simulink model "DC_motor_trans_fcn_25_04"  (R2020b)
settings: Solver=VariableStepAuto  StartTime=0.0  StopTime=10.0  RelTol=1e-3
undefined symbols (not defined in the file or in its folder): B, J, K, L, R
libraries: simulink_extras x1
settings Model: Creator=ADHIP  LastModifiedBy=ADHIP

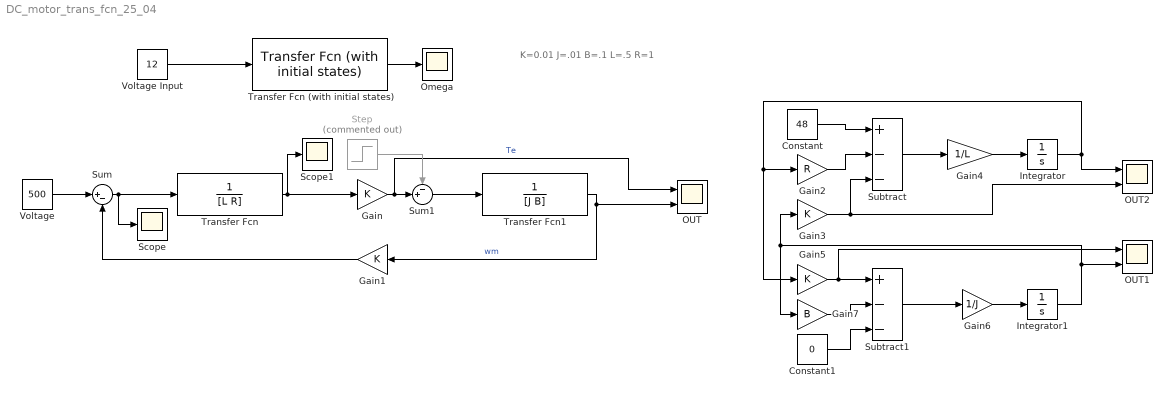
== system DC_motor_trans_fcn_25_04 ==
  note: K=0.01
      | J=.01
      | B=.1
      | L=.5
      | R=1
  Constant : Constant  Value=48
  Constant1 : Constant  Value=0
  Gain{,1,3,5} (4 alike) : Gain  Gain=K
  Gain2 : Gain  Gain=R
  Gain4 : Gain  Gain=1/L
  Gain6 : Gain  Gain=1/J
  Gain7 : Gain  Gain=B
  Integrator : Integrator
  Integrator1 : Integrator
  OUT : Scope  NumInputPorts=2
  OUT1 : Scope  NumInputPorts=2
  OUT2 : Scope  NumInputPorts=2
  Omega : Scope
  Scope : Scope
  Scope1 : Scope
  Step : Step  Commented=on  Time=5  SampleTime=0
  Subtract : Sum  Inputs=+--
  Subtract1 : Sum  Inputs=+--
  Sum : Sum  Inputs=|+-
  Sum1 : Sum  Inputs=-+|
  Transfer Fcn : TransferFcn  Denominator=[L R]
  Transfer Fcn (with initial states) : simulink_extras/Additional Linear/Transfer Fcn (with initial states)  N=[K]  D="[J*L B*L+R*J  B*R+K^2]"  X0=0
  Transfer Fcn1 : TransferFcn  Denominator=[J B]
  Voltage : Constant  Value=500
  Voltage Input : Constant  Value=12
  wires:
  Transfer Fcn (with initial states)/1 -> Omega/1
  Voltage Input/1 -> Transfer Fcn (with initial states)/1
  Voltage/1 -> Sum/1
  Transfer Fcn/1 -> Scope1/1, Gain/1
  Gain1/1 -> Sum/2
  Sum/1 -> Transfer Fcn/1, Scope/1
  Sum1/1 -> Transfer Fcn1/1
  Gain/1 -> OUT/1, Sum1/2  "Te"
  Step/1 -> Sum1/1
  Transfer Fcn1/1 -> OUT/2, Gain1/1  "wm"
  Constant/1 -> Subtract/1
  Gain2/1 -> Subtract/2
  Gain3/1 -> OUT2/2, Subtract/3
  Subtract/1 -> Gain4/1
  Gain4/1 -> Integrator/1
  Integrator/1 -> OUT2/1, Gain2/1, Gain5/1
  Gain5/1 -> OUT1/1, Subtract1/1
  Subtract1/1 -> Gain6/1
  Gain6/1 -> Integrator1/1
  Integrator1/1 -> OUT1/2, Gain7/1, Gain3/1
  Gain7/1 -> Subtract1/2
  Constant1/1 -> Subtract1/3
